simulink library "kif"  (R2022a)
settings: Solver=VariableStepAuto  StartTime=0.0  StopTime=10.0  RelTol=1e-3
undefined symbols (not defined in the file or in its folder): DiscIntNeverNeededParam
libraries: $bdroot x12, spsThreePhaseDynamicLoadLib x4, spsThreePhaseSeriesRLCLoadLib x1, spsGroundLib x1, spsSeriesRLCLoadLib x1, spsControlledCurrentSourceLib x1, spsFourierLib x1, spsPLLLib x1, spsSeriesRLCBranchLib x1, spsVoltageMeasurementLib x1, spsThreePhasePISectionLineLib x1, spsThreePhaseVIMeasurementLib x1
settings Model: Creator=Felhasználó  LastModifiedBy=Felhasználó

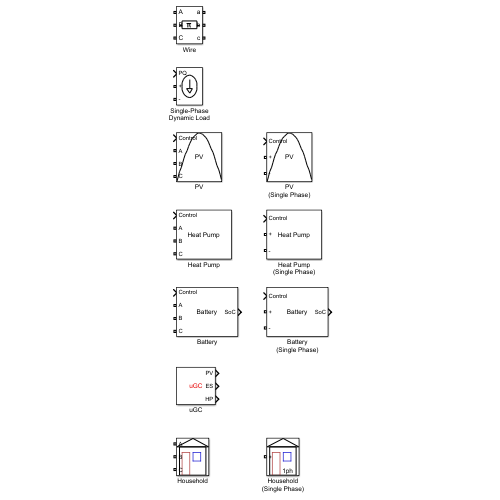
[thumbnail: Simulink's stored preview of the top-level diagram]
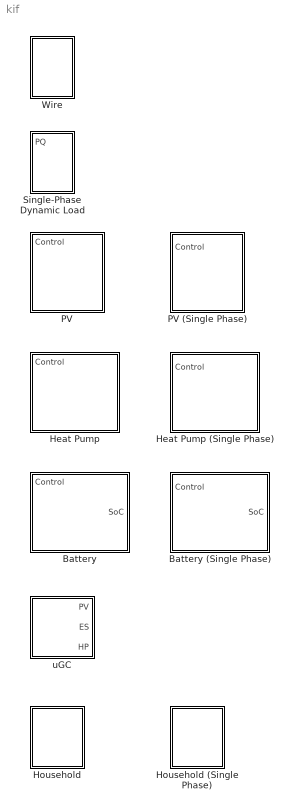
== system kif ==
  Battery : Subsystem  mask(Battery (Three Phase)){Cap=5000, SoCin=0.5, SoCmin=0.2, SoCmax=0.8, Pin=500, eta_in=0.95, Pout=-500, eta_out=0.95, Pmin=0, PQtag=PQ_ESxx, PQtagv=global}
      mask prompts: Cap "Capacity (Wh)"; SoCin "Initial SoC (%)"; SoCmin "Min. SoC (%)"; SoCmax "Max. SoC (%)"; Pin "Max. charging power (W)"; eta_in "Charging efficiency (%)"; Pout "Max. discharging power (W)"; eta_out "Discharging efficiency (%)"; Pmin "Min. power (W)"; PQtag "PQ tag"; PQtagv "Visibility"
      mask help: This block models a battery.
      mask TypeOptions PQtag: Measurement/GotoTag
      mask TypeOptions PQtagv: Measurement/TagVisibility
      mask DialogControl Container3 Prompt: Measurements
      mask Display: disp('Battery');
  Battery (Single Phase) : Subsystem  mask(Battery (Single Phase)){Cap=5000, SoCin=0.5, SoCmin=0.2, SoCmax=0.8, Pin=500, eta_in=0.95, Pout=-500, eta_out=0.95, Pmin=0, PQtag=PQ_ESxx, PGtagv=global}
      mask prompts: Cap "Capacity (Wh)"; SoCin "Initial SoC (%)"; SoCmin "Min. SoC (%)"; SoCmax "Max. SoC (%)"; Pin "Max. charging power (W)"; eta_in "Charging efficiency (%)"; Pout "Max. discharging power (W)"; eta_out "Discharging efficiency (%)"; Pmin "Min. power (W)"; PQtag "PQ tag"; PGtagv "Visibility"
      mask help: This block models a battery.
      mask TypeOptions PQtag: Measurement/GotoTag
      mask TypeOptions PGtagv: Measurement/TagVisibility
      mask DialogControl Container3 Prompt: Measurements
      mask Display: disp('Battery');
  Heat Pump : Subsystem  mask(Heat Pump (Three Phase)){MFSystemSampleTime=0.05, tequiv=3, P_HP=3800, Tset=21, T_init=21, C=5940, H=192, ASHP=on, Mode=on, coeffs=[0.0012, -0.18, 8.6712], T_amb_in=T_amb, PQtag=PQ_HPxx, PQtagv=global}
      mask prompts: MFSystemSampleTime "Simulink:blkprm_prompts:AllBlksSampleTime"; tequiv "Equivalent time (minutes)"; P_HP "Heat pump power (W)"; Tset "Set temperature (°C)"; T_init "Initial Temperature (°C)"; C "Building heat capacity (Wh/K)"; H "Building heat loss coefficient (W/K)"; ASHP "Air source heat pump"; Mode "Heating (/Cooling)"; coeffs "COP coefficients [a2 a1 a0]"; T_amb_in "Ambient temperature input"; PQtag "PQ tag"; PQtagv "Visibility"
      mask help: This block models an SG-Ready AHSP/WSHP/GSHP heat pump.
      mask TypeOptions MFSystemSampleTime: MATLAB Function/SystemSampleTime
      mask TypeOptions T_amb_in: T_amb/GotoTag
      mask TypeOptions PQtag: Measurement/GotoTag
      mask TypeOptions PQtagv: Measurement/TagVisibility
      mask DialogControl MFSystemSampleTime Prompt: Sample time (-1 for inherited):
      mask DialogControl Container3 Prompt: Measurements
      mask Display: disp('Heat Pump');
  Heat Pump (Single Phase) : Subsystem  mask(Heat Pump (Three Phase)){MFSystemSampleTime=0.05, tequiv=3, P_HP=3800, Tset=21, T_init=21, C=5940, H=192, ASHP=on, Mode=on, coeffs=[0.0012, -0.18, 8.6712], T_amb_in=T_amb, PQtag=PQ_HPxx, PQtagv=global}
      mask prompts: MFSystemSampleTime "Simulink:blkprm_prompts:AllBlksSampleTime"; tequiv "Equivalent time (minutes)"; P_HP "Heat pump power (W)"; Tset "Set temperature (°C)"; T_init "Initial Temperature (°C)"; C "Building heat capacity (Wh/K)"; H "Building heat loss coefficient (W/K)"; ASHP "Air source heat pump"; Mode "Heating (/Cooling)"; coeffs "COP coefficients [a2 a1 a0]"; T_amb_in "Ambient temperature input"; PQtag "PQ tag"; PQtagv "Visibility"
      mask help: This block models an SG-Ready AHSP/WSHP/GSHP heat pump.
      mask TypeOptions MFSystemSampleTime: MATLAB Function/SystemSampleTime
      mask TypeOptions T_amb_in: T_amb/GotoTag
      mask TypeOptions PQtag: Measurement/GotoTag
      mask TypeOptions PQtagv: Measurement/TagVisibility
      mask DialogControl MFSystemSampleTime Prompt: Sample time (-1 for inherited):
      mask DialogControl Container3 Prompt: Measurements
      mask Display: disp('Heat Pump');
  Household : Subsystem  mask(Household (Three Phase)){Ctag=CONSxx}
      mask prompts: Ctag "Consumption tag"
      mask help: Represents a household, with PV, battery, heat pump and consumption.
      mask TypeOptions Ctag: Consumption/GotoTag
      mask Display:
      | plot([-5 -5 5 5 -5], [0 10 10 0 0]);
      | plot([-6 0 6 -6], [10 13 10 10]);
      | color('blue');
      | plot([0 3 3 0 0], [5 5 8 8 5]);
      | color('brown');
      | plot([-4 -1 -1 -4 -4], [0 0 8 8 0]);
  Household (Single Phase) : Subsystem  mask(Household (Single Phase)){Ctag=CONSxx}
      mask prompts: Ctag "Consumption tag"
      mask help: Represents a household (single phase), with PV, battery, heat pump and consumption.
      mask TypeOptions Ctag: Consumption/GotoTag
      mask Display:
      | plot([-5 -5 5 5 -5], [0 10 10 0 0]);
      | plot([-6 0 6 -6], [10 13 10 10]);
      | color('blue');
      | plot([0 3 3 0 0], [5 5 8 8 5]);
      | color('brown');
      | plot([-4 -1 -1 -4 -4], [0 0 8 8 0]);
      | color('black')
      | text(0,2, '1ph');
  PV : Subsystem  mask(PV (Three Phase)){P_STCm=2500, Ucoeff=[6.2 26.9], Kcoeff=[0.000005 0.00017 0.000149 -0.004702 -0.040465 -0.017237], IIrradTag=Irrad, T_AmbTag=T_Amb, WindTag=Wind, PQtag=PQ_PVxx, PQtagv=global}
      mask prompts: P_STCm "Peak Power (W)"; Ucoeff "Module temperature coefficients [u1 u0]"; Kcoeff "PV power dependence on irradiance and module temperature [k6 k5 k4 k3 k2 k1]"; IIrradTag "Irradiance input"; T_AmbTag "Ambient temperature input"; WindTag "Wind speed input"; PQtag "PQ tag"; PQtagv "Visibility"
      mask help: This block models a photovoltaic array.
      mask init:
      | U1 = Ucoeff(1);
      |     U0 = Ucoeff(2);
      |     k6 = Kcoeff(1);
      |     k5 = Kcoeff(2);
      |     k4 = Kcoeff(3);
      |     k3 = Kcoeff(4);
      |     k2 = Kcoeff(5);
      |     k1 = Kcoeff(6);
      mask Help: https://joint-research-centre.ec.europa.eu/photovoltaic-geographical-information-system-pvgis/getting-started-pvgis/pvgis-data-sources-calculation-methods_en
      mask TypeOptions IIrradTag: From/GotoTag
      mask TypeOptions T_AmbTag: From1/GotoTag
      mask TypeOptions WindTag: From2/GotoTag
      mask TypeOptions PQtag: Measurement/GotoTag
      mask TypeOptions PQtagv: Measurement/TagVisibility
      mask DialogControl Container3 Prompt: Signal input tags
      mask DialogControl Container4 Prompt: Measurements
      mask Display:
      | disp('PV');
      | 
      | plot(-pi/2:0.1:pi/2, cos(-pi/2:0.1:pi/2));
  PV (Single Phase) : Subsystem  mask(PV (Three Phase)){P_STCm=2500, Ucoeff=[6.2 26.9], Kcoeff=[0.000005 0.00017 0.000149 -0.004702 -0.040465 -0.017237], IIrradTag=Irrad, T_AmbTag=T_Amb, WindTag=Wind, PQtag=PQ_PVxx, PQtagv=global}
      mask prompts: P_STCm "Peak Power (W)"; Ucoeff "Module temperature coefficients [u1 u0]"; Kcoeff "PV power dependence on irradiance and module temperature [k6 k5 k4 k3 k2 k1]"; IIrradTag "Irradiance input"; T_AmbTag "Ambient temperature input"; WindTag "Wind speed input"; PQtag "PQ tag"; PQtagv "Visibility"
      mask help: This block models a photovoltaic array.
      mask init:
      | U1 = Ucoeff(1);
      |     U0 = Ucoeff(2);
      |     k6 = Kcoeff(1);
      |     k5 = Kcoeff(2);
      |     k4 = Kcoeff(3);
      |     k3 = Kcoeff(4);
      |     k2 = Kcoeff(5);
      |     k1 = Kcoeff(6);
      mask Help: https://joint-research-centre.ec.europa.eu/photovoltaic-geographical-information-system-pvgis/getting-started-pvgis/pvgis-data-sources-calculation-methods_en
      mask TypeOptions IIrradTag: From/GotoTag
      mask TypeOptions T_AmbTag: From1/GotoTag
      mask TypeOptions WindTag: From2/GotoTag
      mask TypeOptions PQtag: Measurement/GotoTag
      mask TypeOptions PQtagv: Measurement/TagVisibility
      mask DialogControl Container3 Prompt: Signal input tags
      mask DialogControl Container4 Prompt: Measurements
      mask Display:
      | disp('PV');
      | 
      | plot(-pi/2:0.1:pi/2, cos(-pi/2:0.1:pi/2));
  Single-Phase Dynamic Load : Subsystem  mask(Single-Phase Dynamic Load){Freq=50}
      mask prompts: Freq "Fundamental frequency (Hz):"
      mask help: This block models a PQ controlled single phase dynamic load.
      mask TypeOptions Freq: Fourier/Freq
      mask DialogControl ParameterGroupVar Prompt: PLL
      mask Display:
      | plot(-45,-45,45,45,[0,9,18,24,29,30,29,24,18,9,0,-9,-18,-24,-29,-30,-29,-24,-18,-9,0]*.9,[30,29,24,18,9,0,-9,-18,-24,-29,-30,-29,-24,-18,-9,0,9,18,24,29,30]*.9)
      | plot([0,0,10,0,-10,0]*1.1,[15,-5,-5,-15,-5,-5]*1.1)
  Wire : Subsystem  mask(Three-Phase Low Voltage Distribution Line){Length=0.03, Frequency=50, Resistances=[0.2968 0.4468], Inductances=[0.95359e-3  5.4671e-3], Capacitances=[12.458e-9 3.9055e-9], Vtag=V_Lxx, Vtagv=global, Itag=I_Lxx, Itagv=global}
      mask prompts: Length "Line length (km):"; Frequency "Frequency used for rlc specification (Hz):"; Resistances "Positive- and zero-sequence resistances (Ohms/km) [ r1  r0 ]:"; Inductances "Positive- and zero-sequence inductances (H/km) [ l1  l0 ]:"; Capacitances "Positive- and zero-sequence capacitances (F/km) [ c1 c0 ]:"; Vtag "V tag"; Vtagv "Visibility"; Itag "I tag"; Itagv "Visibility"
      mask help: This block models a low voltage distribution line with a Three-Phase PI Section Line, corresponding ports and V-I measurement.
      mask TypeOptions Length:
      | Three-Phase
      | PI Section Line/Length
      mask TypeOptions Frequency:
      | Three-Phase
      | PI Section Line/Frequency
      mask TypeOptions Resistances:
      | Three-Phase
      | PI Section Line/Resistances
      mask TypeOptions Inductances:
      | Three-Phase
      | PI Section Line/Inductances
      mask TypeOptions Capacitances:
      | Three-Phase
      | PI Section Line/Capacitances
      mask TypeOptions Vtag: Vmeas/GotoTag
      mask TypeOptions Vtagv: Vmeas/TagVisibility
      mask TypeOptions Itag: Imeas/GotoTag
      mask TypeOptions Itagv: Imeas/TagVisibility
      mask DialogControl Container3 Prompt: Measurements
      mask Display: block_icon('Three-Phase PI Section Line');
  uGC : Subsystem  mask(Microgrid Controller){fromCONS=CONSxx, fromPV=PQ_PVxx, fromHP=PQ_HPxx, fromAGGR=Signal}
      mask prompts: fromCONS "Consumption"; fromPV "PV"; fromHP "Heat Pump"; fromAGGR "Aggregator Signal"
      mask help: This block models a microgrid controller. It accepts aggregator signals, and controls PV, battery and heat pump.
      mask TypeOptions fromCONS: From Consumption/GotoTag
      mask TypeOptions fromPV: From PV/GotoTag
      mask TypeOptions fromHP: From Heat Pump/GotoTag
      mask TypeOptions fromAGGR: From Aggregator/GotoTag
      mask Display:
      | color('red');
      | disp('uGC');

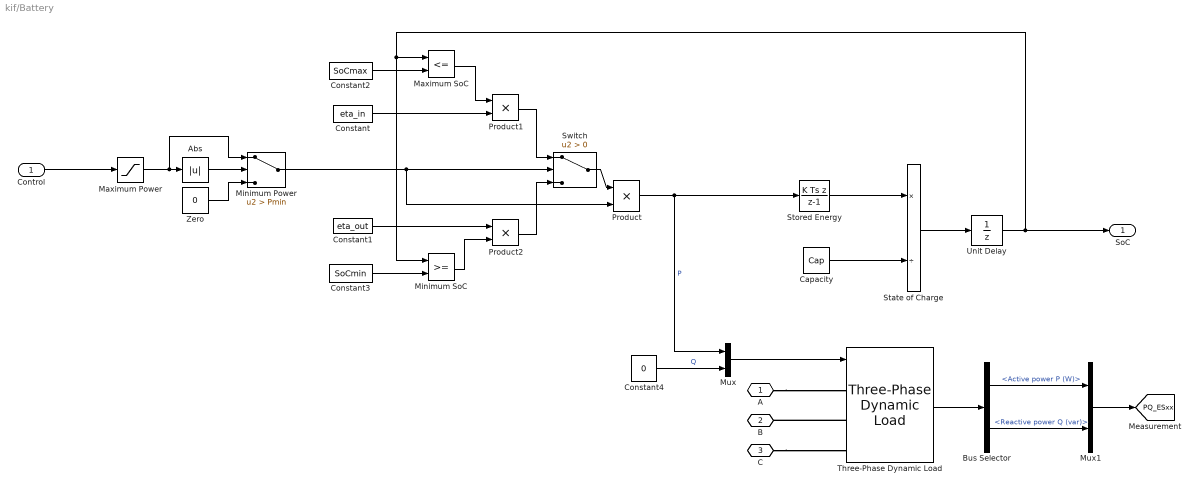
== system kif/Battery ==
  Control : Inport
  Abs : Abs  SaturateOnIntegerOverflow=off
  Bus Selector : BusSelector  OutputSignals=Active power P (W),Reactive power Q (var)
  Capacity : Constant  Value=Cap
  Constant : Constant  Value=eta_in
  Constant1 : Constant  Value=eta_out
  Constant2 : Constant  Value=SoCmax
  Constant3 : Constant  Value=SoCmin
  Constant4 : Constant  Value=0
  Maximum Power : Saturate  UpperLimit=Pin  LowerLimit=Pout
  Maximum SoC : RelationalOperator  Operator=<=  OutDataTypeStr=boolean  RndMeth=Simplest  InputSameDT=off
  Minimum Power : Switch  Criteria=u2 > Threshold  Threshold=Pmin  SaturateOnIntegerOverflow=off  InputSameDT=off
  Minimum SoC : RelationalOperator  OutDataTypeStr=boolean  RndMeth=Simplest  InputSameDT=off
  Mux : Mux  Inputs=2
  Mux1 : Mux  Inputs=2
  Product : Product
  Product1 : Product
  Product2 : Product
  State of Charge : Product  Inputs=*/
  Stored Energy : DiscreteIntegrator  IntegratorMethod=Integration: Backward Euler  InitialCondition=Cap*SoCin  SampleTime=1e-4  ICPrevOutput=DiscIntNeverNeededParam  ICPrevScaledInput=DiscIntNeverNeededParam
  Switch : Switch  Criteria=u2 > Threshold  SaturateOnIntegerOverflow=off  InputSameDT=off
  Three-Phase Dynamic Load : spsThreePhaseDynamicLoadLib/Three-Phase Dynamic Load  NominalVoltage=[ 400 50 ]  ActiveReactivePowers=[0 0]  PositiveSequence=[0.994 -11.8]  ExternalControl=on  NpNq=[1.3 2]  TimeConstants="[0  0  0  0]"  MinimumVoltage=0.7  Tfilter=1e-4  LoadFlowParameters=[4,0,0,0,0]
      settings: SourceProductBaseCode=PS
  Unit Delay : UnitDelay  SampleTime=-1  HasFrameUpgradeWarning=on
  Zero : Constant  Value=0  OutDataTypeStr=Inherit: Inherit via back propagation
  A : PMIOPort  Side=Left
  B : PMIOPort  Port=2  Side=Left
  C : PMIOPort  Port=3  Side=Left
  SoC : Outport
  tag scope: PQ_ESxx=global
  wires:
  Bus Selector/1 -> Mux1/1  "<Active power P (W)>"
  Control/1 -> Maximum Power/1
  Unit Delay/1 -> SoC/1, Minimum SoC/1, Maximum SoC/1
  Constant1/1 -> Product2/1
  Bus Selector/2 -> Mux1/2  "<Reactive power Q (var)>"
  Mux/1 -> Three-Phase Dynamic Load/1
  Switch/1 -> Product/1
  Product/1 -> Mux/1, Stored Energy/1  "P"
  Zero/1 -> Minimum Power/3
  Maximum Power/1 -> Minimum Power/1, Abs/1
  Constant4/1 -> Mux/2  "Q"
  Three-Phase Dynamic Load/1 -> Bus Selector/1
  Minimum Power/1 -> Product/2, Switch/2
  Constant/1 -> Product1/2
  State of Charge/1 -> Unit Delay/1
  Maximum SoC/1 -> Product1/1
  Constant2/1 -> Maximum SoC/2
  Stored Energy/1 -> State of Charge/1
  Product1/1 -> Switch/1
  Capacity/1 -> State of Charge/2
  Abs/1 -> Minimum Power/2
  Product2/1 -> Switch/3
  Minimum SoC/1 -> Product2/2
  Constant3/1 -> Minimum SoC/2
  Mux1/1 -> [PQ_ESxx]
  connections:
  A/RConn1 -- Three-Phase Dynamic Load/LConn1
  C/RConn1 -- Three-Phase Dynamic Load/LConn3
  Three-Phase Dynamic Load/LConn2 -- B/RConn1

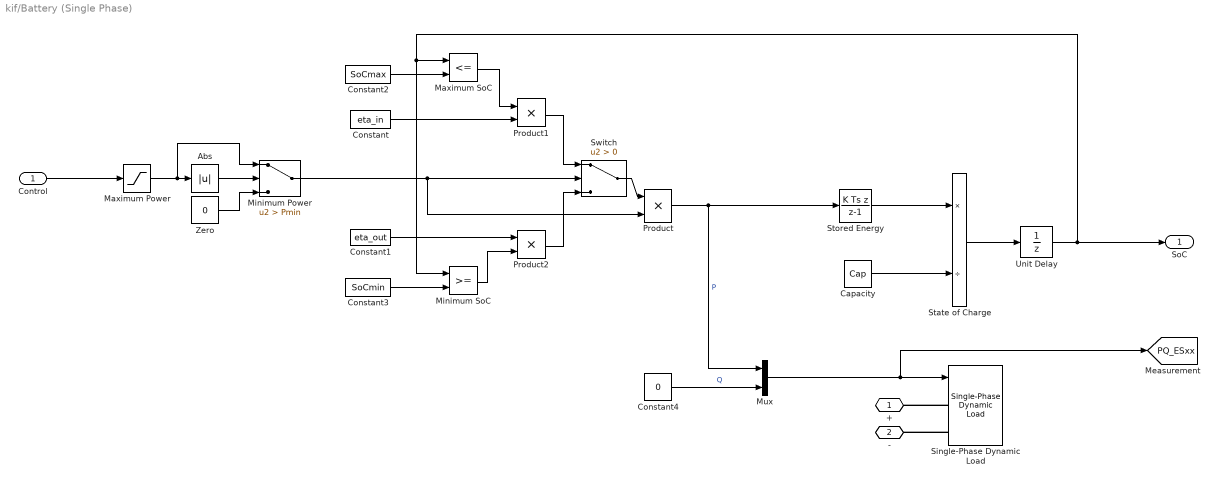
== system kif/Battery (Single Phase) ==
  Control : Inport
  Abs : Abs  SaturateOnIntegerOverflow=off
  Capacity : Constant  Value=Cap
  Constant : Constant  Value=eta_in
  Constant1 : Constant  Value=eta_out
  Constant2 : Constant  Value=SoCmax
  Constant3 : Constant  Value=SoCmin
  Constant4 : Constant  Value=0
  Maximum Power : Saturate  UpperLimit=Pin  LowerLimit=Pout
  Maximum SoC : RelationalOperator  Operator=<=  OutDataTypeStr=boolean  RndMeth=Simplest  InputSameDT=off
  Minimum Power : Switch  Criteria=u2 > Threshold  Threshold=Pmin  SaturateOnIntegerOverflow=off  InputSameDT=off
  Minimum SoC : RelationalOperator  OutDataTypeStr=boolean  RndMeth=Simplest  InputSameDT=off
  Mux : Mux  Inputs=2
  Product : Product
  Product1 : Product
  Product2 : Product
  Single-Phase Dynamic Load : $bdroot/Single-Phase Dynamic Load  Freq=50
  State of Charge : Product  Inputs=*/
  Stored Energy : DiscreteIntegrator  IntegratorMethod=Integration: Backward Euler  InitialCondition=Cap*SoCin  SampleTime=1e-4  ICPrevOutput=DiscIntNeverNeededParam  ICPrevScaledInput=DiscIntNeverNeededParam
  Switch : Switch  Criteria=u2 > Threshold  SaturateOnIntegerOverflow=off  InputSameDT=off
  Unit Delay : UnitDelay  SampleTime=-1  HasFrameUpgradeWarning=on
  Zero : Constant  Value=0  OutDataTypeStr=Inherit: Inherit via back propagation
  + : PMIOPort  Side=Left
  - : PMIOPort  Port=2  Side=Left
  SoC : Outport
  tag scope: PQ_ESxx=global
  wires:
  Control/1 -> Maximum Power/1
  Unit Delay/1 -> SoC/1, Minimum SoC/1, Maximum SoC/1
  Constant1/1 -> Product2/1
  Switch/1 -> Product/1
  Product/1 -> Mux/1, Stored Energy/1  "P"
  Zero/1 -> Minimum Power/3
  Maximum Power/1 -> Minimum Power/1, Abs/1
  Constant4/1 -> Mux/2  "Q"
  Minimum Power/1 -> Product/2, Switch/2
  Constant/1 -> Product1/2
  State of Charge/1 -> Unit Delay/1
  Maximum SoC/1 -> Product1/1
  Constant2/1 -> Maximum SoC/2
  Stored Energy/1 -> State of Charge/1
  Product1/1 -> Switch/1
  Capacity/1 -> State of Charge/2
  Abs/1 -> Minimum Power/2
  Product2/1 -> Switch/3
  Minimum SoC/1 -> Product2/2
  Constant3/1 -> Minimum SoC/2
  Mux/1 -> Single-Phase Dynamic Load/1, [PQ_ESxx]
  connections:
  Single-Phase Dynamic Load/LConn1 -- +/RConn1
  Single-Phase Dynamic Load/LConn2 -- -/RConn1

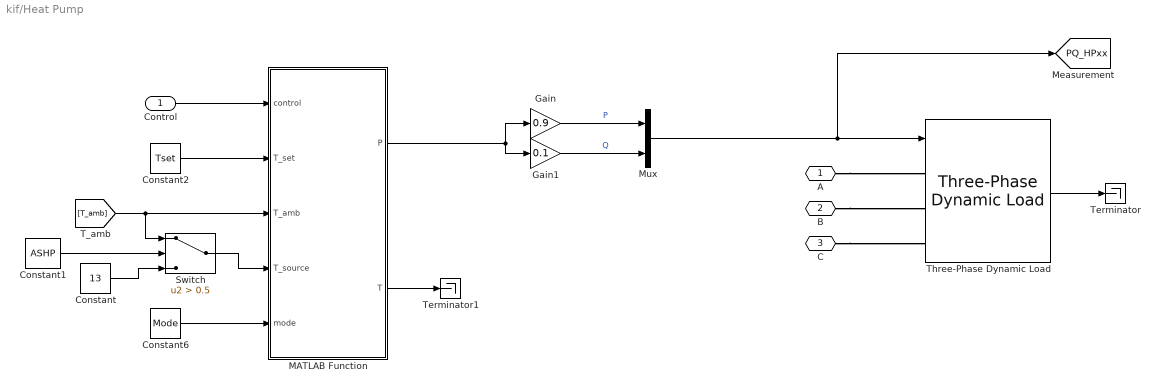
== system kif/Heat Pump ==
  Control : Inport
  Constant : Constant  Value=13
  Constant1 : Constant  Value=ASHP
  Constant2 : Constant  Value=Tset
  Constant6 : Constant  Value=Mode
  Gain : Gain  Gain=0.9
  Gain1 : Gain  Gain=0.1
  MATLAB Function : MATLAB Function  TreatAsAtomicUnit=on  SystemSampleTime=MFSystemSampleTime
  Mux : Mux  Inputs=2
  Switch : Switch  Criteria=u2 > Threshold  Threshold=0.5  SaturateOnIntegerOverflow=off  InputSameDT=off
  Terminator : Terminator
  Terminator1 : Terminator
  Three-Phase Dynamic Load : spsThreePhaseDynamicLoadLib/Three-Phase Dynamic Load  NominalVoltage=[ 400 50 ]  ActiveReactivePowers=[0 0]  PositiveSequence=[0.994 -11.8]  ExternalControl=on  NpNq=[1.3 2]  TimeConstants="[0  0  0  0]"  MinimumVoltage=0.7  Tfilter=1e-4  LoadFlowParameters=[4,0,0,0,0]
      settings: SourceProductBaseCode=PS
  A : PMIOPort  Side=Left
  B : PMIOPort  Port=2  Side=Left
  C : PMIOPort  Port=3  Side=Left
  tag scope: PQ_HPxx=global
  wires:
  MATLAB Function/1(P) -> Gain1/1, Gain/1
  Gain1/1 -> Mux/2  "Q"
  Three-Phase Dynamic Load/1 -> Terminator/1
  Gain/1 -> Mux/1  "P"
  Mux/1 -> [PQ_HPxx], Three-Phase Dynamic Load/1
  [T_amb] -> Switch/1, MATLAB Function/3(T_amb)
  Constant2/1 -> MATLAB Function/2(T_set)
  Constant6/1 -> MATLAB Function/5(mode)
  Constant/1 -> Switch/3
  Switch/1 -> MATLAB Function/4(T_source)
  Constant1/1 -> Switch/2
  Control/1 -> MATLAB Function/1(control)
  MATLAB Function/2(T) -> Terminator1/1
  connections:
  C/RConn1 -- Three-Phase Dynamic Load/LConn3
  B/RConn1 -- Three-Phase Dynamic Load/LConn2
  A/RConn1 -- Three-Phase Dynamic Load/LConn1

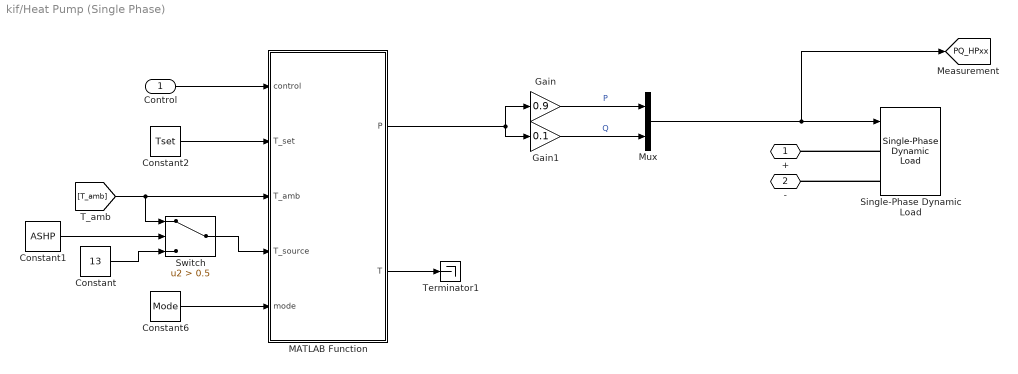
== system kif/Heat Pump (Single Phase) ==
  Control : Inport
  Constant : Constant  Value=13
  Constant1 : Constant  Value=ASHP
  Constant2 : Constant  Value=Tset
  Constant6 : Constant  Value=Mode
  Gain : Gain  Gain=0.9
  Gain1 : Gain  Gain=0.1
  MATLAB Function : MATLAB Function  TreatAsAtomicUnit=on  SystemSampleTime=MFSystemSampleTime
  Mux : Mux  Inputs=2
  Single-Phase Dynamic Load : $bdroot/Single-Phase Dynamic Load  Freq=50
  Switch : Switch  Criteria=u2 > Threshold  Threshold=0.5  SaturateOnIntegerOverflow=off  InputSameDT=off
  Terminator1 : Terminator
  + : PMIOPort  Side=Left
  - : PMIOPort  Port=2  Side=Left
  tag scope: PQ_HPxx=global
  wires:
  MATLAB Function/1(P) -> Gain1/1, Gain/1
  Gain1/1 -> Mux/2  "Q"
  Gain/1 -> Mux/1  "P"
  [T_amb] -> Switch/1, MATLAB Function/3(T_amb)
  Constant2/1 -> MATLAB Function/2(T_set)
  Constant6/1 -> MATLAB Function/5(mode)
  Constant/1 -> Switch/3
  Switch/1 -> MATLAB Function/4(T_source)
  Constant1/1 -> Switch/2
  Control/1 -> MATLAB Function/1(control)
  MATLAB Function/2(T) -> Terminator1/1
  Mux/1 -> Single-Phase Dynamic Load/1, [PQ_HPxx]
  connections:
  Single-Phase Dynamic Load/LConn1 -- +/RConn1
  Single-Phase Dynamic Load/LConn2 -- -/RConn1

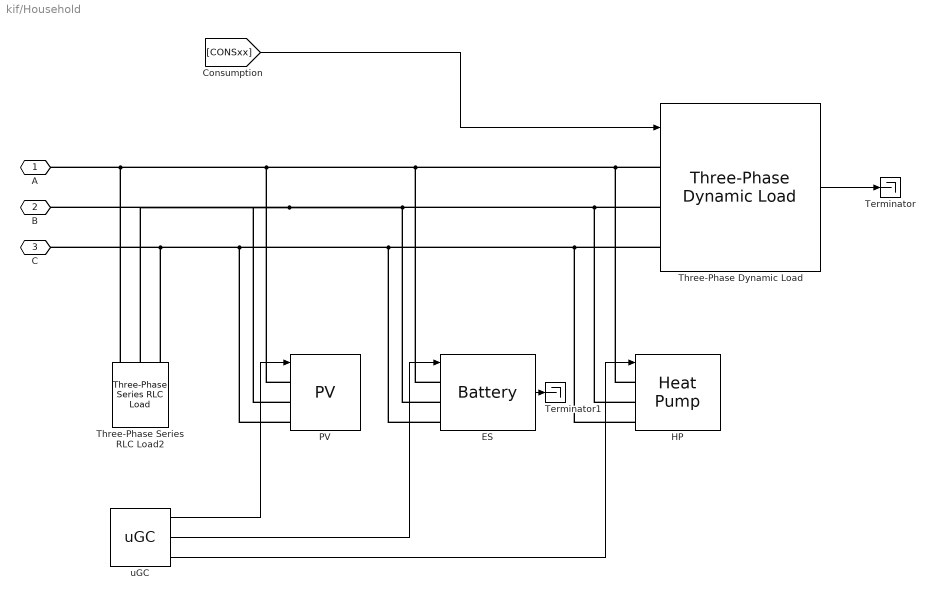
== system kif/Household ==
  ES : $bdroot/Battery  Cap=5000  SoCin=0.5  SoCmin=0.2  SoCmax=0.8  Pin=500  eta_in=0.95  Pout=-500  eta_out=0.95  Pmin=100  PQtag=PQ_ESxx  PQtagv=global
  HP : $bdroot/Heat Pump  MFSystemSampleTime=0.05  tequiv=3  P_HP=3800  Tset=21  T_init=21  C=5940  H=192  ASHP=on  Mode=on  coeffs=[0.0012, -0.18, 8.6712]  T_amb_in=T_amb  PQtag=PQ_HPxx  PQtagv=global
  PV : $bdroot/PV  P_STCm=2500  Ucoeff=[6.2 26.9]  Kcoeff=[0.000005 0.00017 0.000149 -0.004702 -0.040465 -0.017237]  IIrradTag=Irrad  T_AmbTag=T_Amb  WindTag=Wind  PQtag=PQ_PVxx  PQtagv=global
  Terminator : Terminator
  Terminator1 : Terminator
  Three-Phase Dynamic Load : spsThreePhaseDynamicLoadLib/Three-Phase Dynamic Load  NominalVoltage=[ 400 50 ]  ActiveReactivePowers=[0 0]  PositiveSequence=[0.994 -11.8]  ExternalControl=on  NpNq=[1.3 2]  TimeConstants="[0  0  0  0]"  MinimumVoltage=0.7  Tfilter=1e-4  LoadFlowParameters=[4,0,0,0,0]
      settings: SourceProductBaseCode=PS
  Three-Phase Series RLC Load2 : spsThreePhaseSeriesRLCLoadLib/Three-Phase Series RLC Load  LConnTagsString=A|B|C  Configuration=Y (grounded)  NominalVoltage=400  Vabc=[1e3 1e3 1e3]  Vabcp=[1e3 1e3 1e3]  NominalFrequency=50  UnbalancedPower=off  ActivePower=1  InductivePower=0  CapacitivePower=0  Pabc=[10e3 9e3 11e3]  QLabc=[100 90 110]  QCabc=[100 90 110]  Pabcp=[10e3 9e3 11e3]  QLabcp=[100 90 110]  QCabcp=[100 90 110]  Measurements=None  LoadType=constant Z
  uGC : $bdroot/uGC  fromCONS=CONSxx  fromPV=PQ_PVxx  fromHP=PQ_HPxx  fromAGGR=Signal
  A : PMIOPort  Side=Left
  B : PMIOPort  Port=2  Side=Left
  C : PMIOPort  Port=3  Side=Left
  wires:
  uGC/1 -> PV/1
  Three-Phase Dynamic Load/1 -> Terminator/1
  ES/1 -> Terminator1/1
  uGC/3 -> HP/1
  uGC/2 -> ES/1
  [CONSxx] -> Three-Phase Dynamic Load/1
  connections:
  Three-Phase Dynamic Load/LConn1 -- HP/LConn1 -- ES/LConn1 -- PV/LConn1 -- A/RConn1 -- Three-Phase Series RLC Load2/LConn1
  Three-Phase Dynamic Load/LConn2 -- HP/LConn2 -- B/RConn1 -- Three-Phase Series RLC Load2/LConn2 -- PV/LConn2 -- ES/LConn2
  Three-Phase Dynamic Load/LConn3 -- HP/LConn3 -- PV/LConn3 -- C/RConn1 -- Three-Phase Series RLC Load2/LConn3 -- ES/LConn3

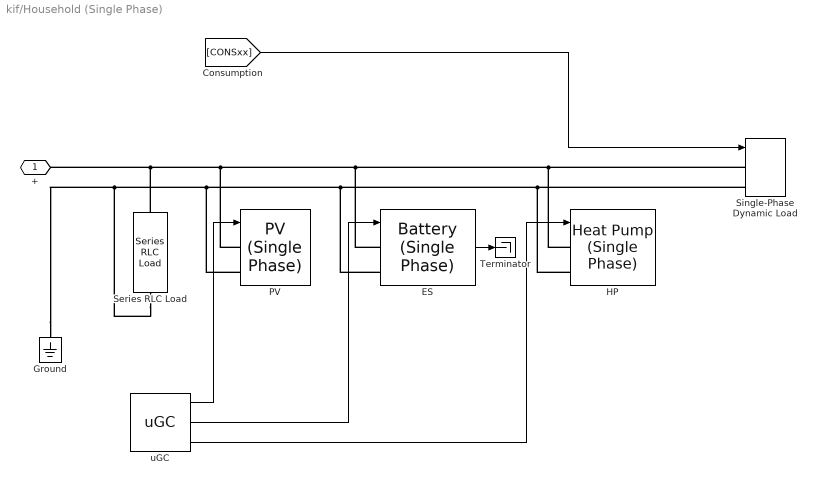
== system kif/Household (Single Phase) ==
  ES : $bdroot/Battery (Single Phase)  Cap=5000  SoCin=0.5  SoCmin=0.2  SoCmax=0.8  Pin=500  eta_in=0.95  Pout=-500  eta_out=0.95  Pmin=100  PQtag=PQ_ESxx  PGtagv=global
  Ground : spsGroundLib/Ground  LConnTagsString=a
  HP : $bdroot/Heat Pump (Single Phase)  MFSystemSampleTime=0.05  tequiv=3  P_HP=3800  Tset=21  T_init=21  C=5940  H=192  ASHP=on  Mode=on  coeffs=[0.0012, -0.18, 8.6712]  T_amb_in=T_amb  PQtag=PQ_HPxx  PQtagv=global
  PV : $bdroot/PV (Single Phase)  P_STCm=2500  Ucoeff=[6.2 26.9]  Kcoeff=[0.000005 0.00017 0.000149 -0.004702 -0.040465 -0.017237]  IIrradTag=Irrad  T_AmbTag=T_Amb  WindTag=Wind  PQtag=PQ_PVxx  PQtagv=global
  Series RLC Load : spsSeriesRLCLoadLib/Series RLC Load  LConnTagsString=a  RConnTagsString=__new0  NominalVoltage=400  NominalFrequency=50  ActivePower=1  InductivePower=0  CapacitivePower=0  Setx0=off  InitialVoltage=0  SetiL0=off  InitialCurrent=0  Measurements=None  LoadType=constant Z
  Single-Phase Dynamic Load : $bdroot/Single-Phase Dynamic Load  Freq=50
  Terminator : Terminator
  uGC : $bdroot/uGC  fromCONS=CONSxx  fromPV=PQ_PVxx  fromHP=PQ_HPxx  fromAGGR=Signal
  + : PMIOPort  Side=Left
  wires:
  [CONSxx] -> Single-Phase Dynamic Load/1
  uGC/1 -> PV/1
  uGC/2 -> ES/1
  ES/1 -> Terminator/1
  uGC/3 -> HP/1
  connections:
  HP/LConn1 -- Single-Phase Dynamic Load/LConn1 -- ES/LConn1 -- PV/LConn1 -- +/RConn1 -- Series RLC Load/LConn1
  Ground/LConn1 -- Single-Phase Dynamic Load/LConn2 -- HP/LConn2 -- ES/LConn2 -- PV/LConn2 -- Series RLC Load/RConn1

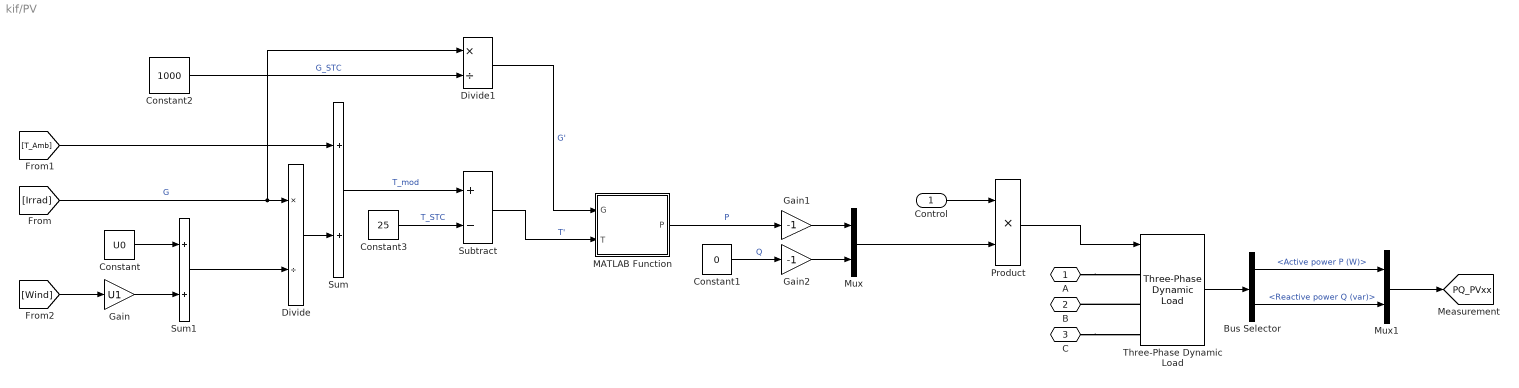
== system kif/PV ==
  Control : Inport
  Bus Selector : BusSelector  OutputSignals=Active power P (W),Reactive power Q (var)
  Constant : Constant  Value=U0
  Constant1 : Constant  Value=0
  Constant2 : Constant  Value=1000
  Constant3 : Constant  Value=25
  Divide : Product  Inputs=*/
  Divide1 : Product  Inputs=*/
  Gain : Gain  Gain=U1
  Gain1 : Gain  Gain=-1
  Gain2 : Gain  Gain=-1
  MATLAB Function : MATLAB Function  TreatAsAtomicUnit=on
  Mux : Mux  Inputs=2
  Mux1 : Mux  Inputs=2
  Product : Product
  Subtract : Sum  Inputs=+-
  Sum : Sum
  Sum1 : Sum
  Three-Phase Dynamic Load : spsThreePhaseDynamicLoadLib/Three-Phase Dynamic Load  NominalVoltage=[ 400 50 ]  ActiveReactivePowers=[0 0]  PositiveSequence=[0.994 -11.8]  ExternalControl=on  NpNq=[1.3 2]  TimeConstants="[0  0  0  0]"  MinimumVoltage=0.7  Tfilter=1e-4  LoadFlowParameters=[4,0,0,0,0]
      settings: SourceProductBaseCode=PS
  A : PMIOPort  Side=Left
  B : PMIOPort  Port=2  Side=Left
  C : PMIOPort  Port=3  Side=Left
  tag scope: PQ_PVxx=global
  wires:
  Constant2/1 -> Divide1/2  "G_STC"
  [Wind] -> Gain/1
  Bus Selector/2 -> Mux1/2  "<Reactive power Q (var)>"
  [Irrad] -> Divide/1, Divide1/1  "G"
  [T_Amb] -> Sum/1
  Constant3/1 -> Subtract/2  "T_STC"
  Sum/1 -> Subtract/1  "T_mod"
  Divide1/1 -> MATLAB Function/1(G)  "G'"
  Constant/1 -> Sum1/1
  Gain/1 -> Sum1/2
  Divide/1 -> Sum/2
  Sum1/1 -> Divide/2
  Subtract/1 -> MATLAB Function/2(T)  "T'"
  MATLAB Function/1(P) -> Gain1/1  "P"
  Constant1/1 -> Gain2/1  "Q"
  Three-Phase Dynamic Load/1 -> Bus Selector/1
  Bus Selector/1 -> Mux1/1  "<Active power P (W)>"
  Control/1 -> Product/1
  Gain1/1 -> Mux/1
  Gain2/1 -> Mux/2
  Mux1/1 -> [PQ_PVxx]
  Mux/1 -> Product/2
  Product/1 -> Three-Phase Dynamic Load/1
  connections:
  Three-Phase Dynamic Load/LConn2 -- B/RConn1
  C/RConn1 -- Three-Phase Dynamic Load/LConn3
  A/RConn1 -- Three-Phase Dynamic Load/LConn1

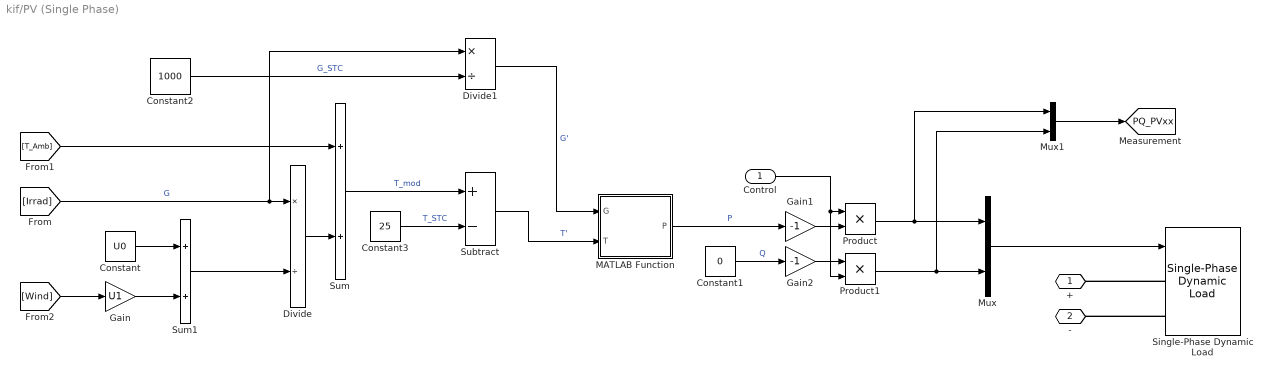
== system kif/PV (Single Phase) ==
  Control : Inport
  Constant : Constant  Value=U0
  Constant1 : Constant  Value=0
  Constant2 : Constant  Value=1000
  Constant3 : Constant  Value=25
  Divide : Product  Inputs=*/
  Divide1 : Product  Inputs=*/
  Gain : Gain  Gain=U1
  Gain1 : Gain  Gain=-1
  Gain2 : Gain  Gain=-1
  MATLAB Function : MATLAB Function  TreatAsAtomicUnit=on
  Mux : Mux  Inputs=2
  Mux1 : Mux  Inputs=2
  Product : Product
  Product1 : Product
  Single-Phase Dynamic Load : $bdroot/Single-Phase Dynamic Load  Freq=50
  Subtract : Sum  Inputs=+-
  Sum : Sum
  Sum1 : Sum
  + : PMIOPort  Side=Left
  - : PMIOPort  Port=2  Side=Left
  tag scope: PQ_PVxx=global
  wires:
  Constant2/1 -> Divide1/2  "G_STC"
  [Wind] -> Gain/1
  [Irrad] -> Divide/1, Divide1/1  "G"
  [T_Amb] -> Sum/1
  Constant3/1 -> Subtract/2  "T_STC"
  Sum/1 -> Subtract/1  "T_mod"
  Divide1/1 -> MATLAB Function/1(G)  "G'"
  Constant/1 -> Sum1/1
  Gain/1 -> Sum1/2
  Divide/1 -> Sum/2
  Sum1/1 -> Divide/2
  Subtract/1 -> MATLAB Function/2(T)  "T'"
  MATLAB Function/1(P) -> Gain1/1  "P"
  Constant1/1 -> Gain2/1  "Q"
  Mux/1 -> Single-Phase Dynamic Load/1
  Mux1/1 -> [PQ_PVxx]
  Gain1/1 -> Product/2
  Product/1 -> Mux/1, Mux1/1
  Gain2/1 -> Product1/1
  Product1/1 -> Mux/2, Mux1/2
  Control/1 -> Product1/2, Product/1
  connections:
  Single-Phase Dynamic Load/LConn1 -- +/RConn1
  Single-Phase Dynamic Load/LConn2 -- -/RConn1

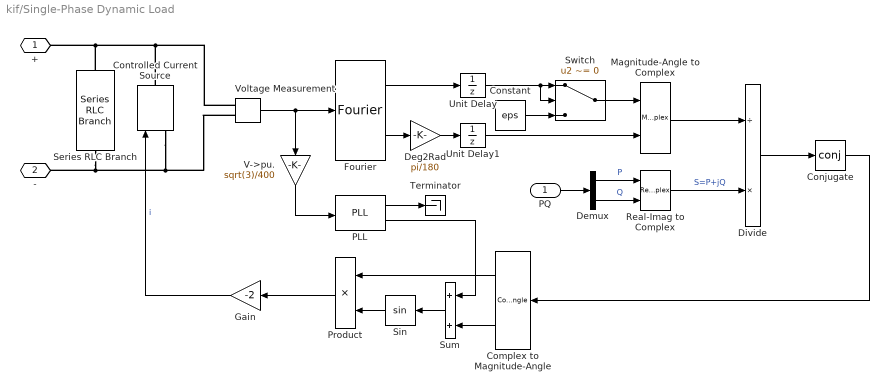
== system kif/Single-Phase Dynamic Load ==
  PQ : Inport
  Complex to Magnitude-Angle : ComplexToMagnitudeAngle
  Conjugate : Math  Operator=conj  SignedPower=on  RndMeth=Zero
  Constant : Constant  Value=eps
  Controlled Current Source : spsControlledCurrentSourceLib/Controlled Current Source  Initialize=on  Source_Type=AC  Amplitude=0  Phase=0  Frequency=50  Measurements=None
  Deg2Rad : Gain  Gain=pi/180
  Demux : Demux  Outputs=2
  Divide : Product  Inputs=/*
  Fourier : spsFourierLib/Fourier  Freq=Freq  n=1  InInit=[400/sqrt(3), 0]  Ts=0
      settings: SourceProductBaseCode=PS
  Gain : Gain  Gain=-2
  Magnitude-Angle to Complex : MagnitudeAngleToComplex
  PLL : spsPLLLib/PLL  Fmin=45  Par_Init=[0, 50]  ParK=[180, 3200, 1]  TcD=1e-4  MaxRateChangeFreq=12  FilterCutOffFreq=25  Ts=0  AGC=on
      settings: SourceProductBaseCode=PS
  Product : Product
  Real-Imag to Complex : RealImagToComplex
  Series RLC Branch : spsSeriesRLCBranchLib/Series RLC Branch  LConnTagsString=__new0  RConnTagsString=__new0  BranchType=R  Resistance=1e6  Inductance=1e-3  SetiL0=off  InitialCurrent=0  Capacitance=1e-6  Setx0=off  InitialVoltage=0  Measurements=None
  Sin : Trigonometry
  Sum : Sum
  Switch : Switch  Criteria=u2 ~= 0  SaturateOnIntegerOverflow=off  InputSameDT=off
  Terminator : Terminator
  Unit Delay : UnitDelay  SampleTime=-1  HasFrameUpgradeWarning=on
  Unit Delay1 : UnitDelay  SampleTime=-1  HasFrameUpgradeWarning=on
  V->pu. : Gain  Gain=sqrt(3)/400
  Voltage Measurement : spsVoltageMeasurementLib/Voltage Measurement  PhasorSimulation=off  OutputType=Complex  PSBequivalent=0
  + : PMIOPort  Side=Left
  - : PMIOPort  Port=2  Side=Left
  wires:
  Divide/1 -> Conjugate/1
  Fourier/1 -> Unit Delay/1
  Complex to Magnitude-Angle/1 -> Product/1
  Magnitude-Angle to Complex/1 -> Divide/1
  Sum/1 -> Sin/1
  PQ/1 -> Demux/1
  Unit Delay1/1 -> Magnitude-Angle to Complex/2
  Voltage Measurement/1 -> V->pu./1, Fourier/1
  Constant/1 -> Switch/3
  PLL/1 -> Terminator/1
  Demux/1 -> Real-Imag to Complex/1  "P"
  Unit Delay/1 -> Switch/2, Switch/1
  Complex to Magnitude-Angle/2 -> Sum/2
  Sin/1 -> Product/2
  Product/1 -> Gain/1
  Real-Imag to Complex/1 -> Divide/2  "S=P+jQ"
  Fourier/2 -> Deg2Rad/1
  Conjugate/1 -> Complex to Magnitude-Angle/1
  Gain/1 -> Controlled Current Source/1  "i"
  Switch/1 -> Magnitude-Angle to Complex/1
  Demux/2 -> Real-Imag to Complex/2  "Q"
  PLL/2 -> Sum/1
  Deg2Rad/1 -> Unit Delay1/1
  V->pu./1 -> PLL/1
  connections:
  Voltage Measurement/LConn2 -- Controlled Current Source/LConn1 -- -/RConn1 -- Series RLC Branch/RConn1
  Voltage Measurement/LConn1 -- +/RConn1 -- Series RLC Branch/LConn1 -- Controlled Current Source/RConn1

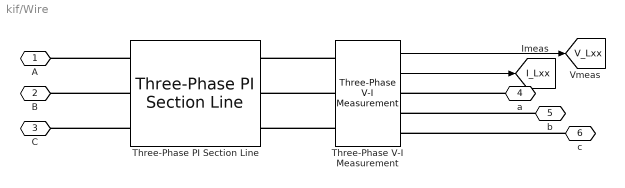
== system kif/Wire ==
  Three-Phase PI Section Line : spsThreePhasePISectionLineLib/Three-Phase PI Section Line  LConnTagsString=a|b|c  RConnTagsString=A|B|C  Length=Length  Frequency=Frequency  Resistances=Resistances  Inductances=Inductances  Capacitances=Capacitances
  Three-Phase V-I Measurement : spsThreePhaseVIMeasurementLib/Three-Phase V-I Measurement  VoltageMeasurement=phase-to-ground  SetLabelV=off  LabelV=Vabc  Vpu=off  VpuLL=off  CurrentMeasurement=yes  SetLabelI=off  LabelI=Iabc  Ipu=off  Pbase=100e6  Vbase=500e3  OutputType=Complex  PhasorSimulation=off  PSBequivalent=0
  A : PMIOPort  Side=Left
  B : PMIOPort  Port=2  Side=Left
  C : PMIOPort  Port=3  Side=Left
  a : PMIOPort  Port=4  Side=Right
  b : PMIOPort  Port=5  Side=Right
  c : PMIOPort  Port=6  Side=Right
  tag scope: I_Lxx=global, V_Lxx=global
  wires:
  Three-Phase V-I Measurement/1 -> [V_Lxx]
  Three-Phase V-I Measurement/2 -> [I_Lxx]
  connections:
  c/RConn1 -- Three-Phase V-I Measurement/RConn3
  Three-Phase PI Section Line/LConn3 -- C/RConn1
  Three-Phase V-I Measurement/LConn3 -- Three-Phase PI Section Line/RConn3
  b/RConn1 -- Three-Phase V-I Measurement/RConn2
  Three-Phase V-I Measurement/LConn2 -- Three-Phase PI Section Line/RConn2
  a/RConn1 -- Three-Phase V-I Measurement/RConn1
  Three-Phase PI Section Line/LConn2 -- B/RConn1
  Three-Phase PI Section Line/LConn1 -- A/RConn1
  Three-Phase V-I Measurement/LConn1 -- Three-Phase PI Section Line/RConn1

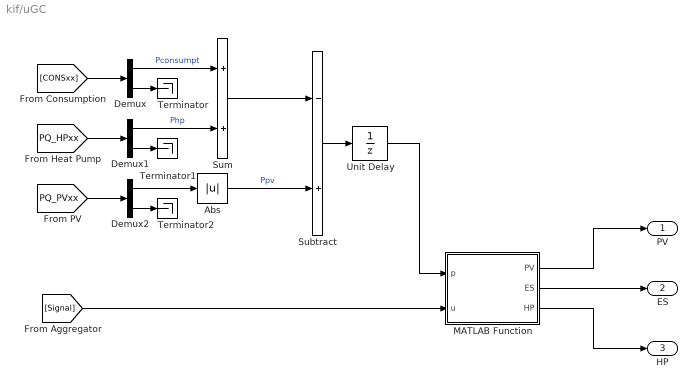
== system kif/uGC ==
  Abs : Abs  SaturateOnIntegerOverflow=off
  Demux : Demux  Outputs=2
  Demux1 : Demux  Outputs=2
  Demux2 : Demux  Outputs=2
  MATLAB Function : MATLAB Function  TreatAsAtomicUnit=on
  Subtract : Sum  Inputs=-+
  Sum : Sum
  Terminator : Terminator
  Terminator1 : Terminator
  Terminator2 : Terminator
  Unit Delay : UnitDelay  SampleTime=-1  HasFrameUpgradeWarning=on
  PV : Outport
  ES : Outport  Port=2
  HP : Outport  Port=3
  wires:
  Sum/1 -> Subtract/1
  Subtract/1 -> Unit Delay/1
  MATLAB Function/3(HP) -> HP/1
  MATLAB Function/1(PV) -> PV/1
  Unit Delay/1 -> MATLAB Function/1(p)
  MATLAB Function/2(ES) -> ES/1
  [CONSxx] -> Demux/1
  Demux/1 -> Sum/1  "Pconsumpt"
  [PQ_HPxx] -> Demux1/1
  [PQ_PVxx] -> Demux2/1
  Demux1/1 -> Sum/2  "Php"
  Demux2/1 -> Abs/1
  Demux/2 -> Terminator/1
  Demux2/2 -> Terminator2/1
  Demux1/2 -> Terminator1/1
  [Signal] -> MATLAB Function/2(u)
  Abs/1 -> Subtract/2  "Ppv"

== matlab function kif/PV/MATLAB Function ==
  data: G input; P output; T input; P_STCm parameter; k1 parameter; k2 parameter; k3 parameter; k4 parameter; k5 parameter; k6 parameter
function P = fcn(G,T, P_STCm, k1, k2, k3, k4, k5, k6)
    if G < eps
        P = 0;
    else
        P = G*(P_STCm + k1*log(G) + k2*log(G)^2 + k3*T + k4*T*log(G) + k5*T*log(G)^2 + k6*T^2);
    end
end

== matlab function kif/PV (Single Phase)/MATLAB Function ==
  data: G input; P output; T input; P_STCm parameter; k1 parameter; k2 parameter; k3 parameter; k4 parameter; k5 parameter; k6 parameter
function P = fcn(G,T, P_STCm, k1, k2, k3, k4, k5, k6)
    if G < eps
        P = 0;
    else
        P = G*(P_STCm + k1*log(G) + k2*log(G)^2 + k3*T + k4*T*log(G) + k5*T*log(G)^2 + k6*T^2);
    end
end

== matlab function kif/Heat Pump (Single Phase)/MATLAB Function ==
  data: P output; control input; T_set input; T_amb input; T_source input; mode input; T output; P_HP parameter; H parameter; C parameter; coeffs parameter; T_init parameter; tequiv parameter
% OFF = 1
% NORMAL = 2
% ON = 3
% SUPERHEAT_A = 4
% SUPERHEAT_B = 5

function [P, T] = fcn(control, T_set, T_amb, T_source, mode, P_HP, H, C, coeffs, T_init, tequiv)
    HYST = 0.5;
    HYST_adj = 1;
    min_run_time = 3;
    min_pause_time = 6;
    T_sink = 45;
    
    persistent pause_time;
    if isempty(pause_time)
        pause_time = 0;
    end
    persistent run_time;
    if isempty(run_time)
        run_time = 0;
    end
    persistent on;
    if isempty(on)
        on = false;
    end
    persistent prev_control;
    if isempty(prev_control)
        prev_control = 2;
    end
    
    persistent T_in;
    if isempty(T_in)
        T_in = T_init;
    end
    
    %initial values
    Q_HP = 0;
    %default hysteresis
    T_min = T_set - HYST;
    T_max = T_set + HYST;
    
    if (mode) %heating
        %adjust histeresis based on control
        if (control == 3 || control >= 4)
            T_min = T_set + HYST_adj;
            T_max = T_set + HYST + HYST_adj;
        end
        %switch on/off
        if (~on && ...
                pause_time >= min_pause_time && ...
                control ~= 1 && ...
                (T_in < T_min || (control >= 4 && prev_control < 4)))
            on = true;
            run_time = 0;
        elseif (on && ...
                run_time >= min_run_time && ...
                (T_in > T_max || control == 1))
            on = false;
            pause_time = 0;
        end
        %determine P and Q
        if (on)
            COP = polyval(coeffs, T_sink - T_source);
            Q_HP = P_HP * COP;
            P = P_HP;
            run_time = run_time + tequiv;
        else
            P = 0;
            pause_time = pause_time + tequiv;
        end
    else %cooling
        %adjust histeresis based on control
        if (control == 3 || control >= 4)
            T_min = T_set - HYST - HYST_adj;
            T_max = T_set - HYST_adj;
        end
        %switch on/off
        if (~on && ...
                pause_time >= min_pause_time && ...
                control ~= 1 && ...
                (T_in > T_max || (control >= 4 && prev_control < 4)))
            on = true;
            run_time = 0;
        elseif (on && ...
                run_time >= min_run_time && ...
                (T_in < T_min || control == 1))
            on = false;
            pause_time = 0;
        end
        %determine P and Q
        if (on)
            COP = polyval(coeffs, T_source - T_sink) - 1;
            Q_HP = - P_HP * COP;
            P = P_HP;
            run_time = run_time + tequiv;
        else
            P = 0;
            pause_time = pause_time + tequiv;
        end
    end
    %simulate diff. eq.
    h = tequiv/60;
    T_in = T_in + h * (-H/C*(T_in - T_amb) + Q_HP/C);
    prev_control = control;
    T = T_in;
end

== matlab function kif/Heat Pump/MATLAB Function ==
  data: P output; control input; T_set input; T_amb input; T_source input; mode input; T output; P_HP parameter; H parameter; C parameter; coeffs parameter; T_init parameter; tequiv parameter
% OFF = 1
% NORMAL = 2
% ON = 3
% SUPERHEAT_A = 4
% SUPERHEAT_B = 5

function [P, T] = fcn(control, T_set, T_amb, T_source, mode, P_HP, H, C, coeffs, T_init, tequiv)
    HYST = 0.5;
    HYST_adj = 1;
    min_run_time = 3;
    min_pause_time = 6;
    T_sink = 45;
    
    persistent pause_time;
    if isempty(pause_time)
        pause_time = 0;
    end
    persistent run_time;
    if isempty(run_time)
        run_time = 0;
    end
    persistent on;
    if isempty(on)
        on = false;
    end
    persistent prev_control;
    if isempty(prev_control)
        prev_control = 2;
    end
    
    persistent T_in;
    if isempty(T_in)
        T_in = T_init;
    end
    
    %initial values
    Q_HP = 0;
    %default hysteresis
    T_min = T_set - HYST;
    T_max = T_set + HYST;
    
    if (mode) %heating
        %adjust histeresis based on control
        if (control == 3 || control >= 4)
            T_min = T_set + HYST_adj;
            T_max = T_set + HYST + HYST_adj;
        end
        %switch on/off
        if (~on && ...
                pause_time >= min_pause_time && ...
                control ~= 1 && ...
                (T_in < T_min || (control >= 4 && prev_control < 4)))
            on = true;
            run_time = 0;
        elseif (on && ...
                run_time >= min_run_time && ...
                (T_in > T_max || control == 1))
            on = false;
            pause_time = 0;
        end
        %determine P and Q
        if (on)
            COP = polyval(coeffs, T_sink - T_source);
            Q_HP = P_HP * COP;
            P = P_HP;
            run_time = run_time + tequiv;
        else
            P = 0;
            pause_time = pause_time + tequiv;
        end
    else %cooling
        %adjust histeresis based on control
        if (control == 3 || control >= 4)
            T_min = T_set - HYST - HYST_adj;
            T_max = T_set - HYST_adj;
        end
        %switch on/off
        if (~on && ...
                pause_time >= min_pause_time && ...
                control ~= 1 && ...
                (T_in > T_max || (control >= 4 && prev_control < 4)))
            on = true;
            run_time = 0;
        elseif (on && ...
                run_time >= min_run_time && ...
                (T_in < T_min || control == 1))
            on = false;
            pause_time = 0;
        end
        %determine P and Q
        if (on)
            COP = polyval(coeffs, T_source - T_sink) - 1;
            Q_HP = - P_HP * COP;
            P = P_HP;
            run_time = run_time + tequiv;
        else
            P = 0;
            pause_time = pause_time + tequiv;
        end
    end
    %simulate diff. eq.
    h = tequiv/60;
    T_in = T_in + h * (-H/C*(T_in - T_amb) + Q_HP/C);
    prev_control = control;
    T = T_in;
end

== matlab function kif/uGC/MATLAB Function ==
  data: p input; u input; PV output; ES output; HP output
function [PV, ES, HP] = fcn(p, u)
    if isnan(p)
        p = 0;
    end
    switch u
        case -1 % down
            PV = 1;
            ES = -inf;
            HP = 1;
        case 0 % normal
            PV = 1;
            ES = p;
            HP = 2;
        case 1 % up
            PV = 0;
            ES = inf;
            HP = 4;
        otherwise % normal
            PV = 1;
            ES = p;
            HP = 2;
    end
end
